simulink subsystem "ElectricMotorcycle"  (R2025b)
settings: Solver=VariableStepAuto  StartTime=0.0  StopTime=10.0  RelTol=1e-3
undefined symbols (not defined in the file): PlntDriveshftDamp, PlntDriveshftStiff, PlntEM1Damp, PlntEM1Inertia, PlntEM1Ratio
libraries: autolibsharedcoupling x2
settings Model: Creator=The MathWorks, Inc.  LastModifiedBy=The MathWorks, Inc.
settings RTWCC: GPUComputeCapability=3.5

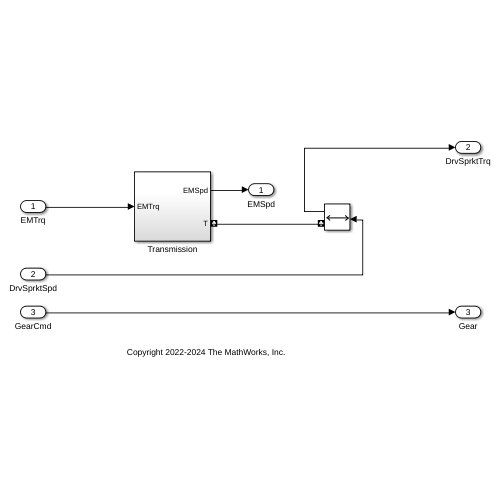
[thumbnail: Simulink's stored preview of the top-level diagram]
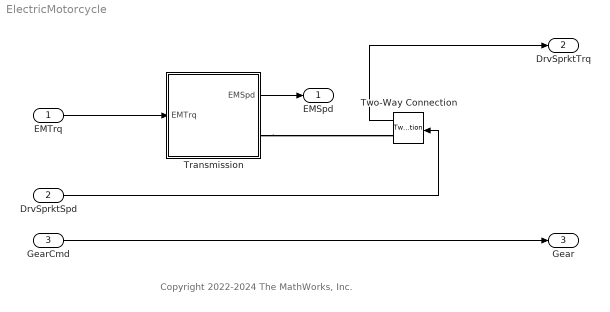
== system ElectricMotorcycle ==
  note: Copyright 2022-2024 The MathWorks, Inc.
  EMTrq : Inport
  DrvSprktSpd : Inport  Port=2
  GearCmd : Inport  Port=3
  Transmission : Subsystem
  Two-Way Connection : TwoWayConnection
  EMSpd : Outport  VectorParamsAs1DForOutWhenUnconnected=off  BusOutputAsStruct=on
  DrvSprktTrq : Outport  Port=2  VectorParamsAs1DForOutWhenUnconnected=off
  Gear : Outport  Port=3
  wires:
  Two-Way Connection/1 -> DrvSprktTrq/1
  Transmission/1(EMSpd) -> EMSpd/1
  EMTrq/1 -> Transmission/1(EMTrq)
  DrvSprktSpd/1 -> Two-Way Connection/1
  GearCmd/1 -> Gear/1
  connections:
  Transmission/RConn1 -- Two-Way Connection/RConn1

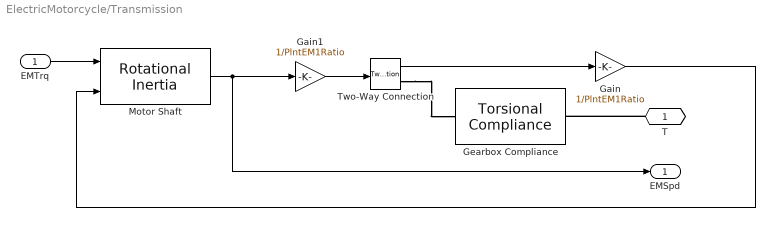
== system ElectricMotorcycle/Transmission ==
  EMTrq : Inport
  Gain : Gain  Gain=1/PlntEM1Ratio
  Gain1 : Gain  Gain=1/PlntEM1Ratio
  Gearbox Compliance : autolibsharedcoupling/Torsional Compliance  port_config=Two-way connection  extInfo=off  k=PlntDriveshftStiff  b=PlntDriveshftDamp  theta_o=PlntDriveshftInitDeflect  domega_o=PlntDriveshftInitVel  omega_c=PlntDriveshftDampCutoffFreq  blkID=0  aMode=6
  Motor Shaft : autolibsharedcoupling/Rotational Inertia  port_config=Simulink  extInfo=off  externJ=off  J=PlntEM1Inertia  b=PlntEM1Damp  omega_o=PlntEM1InitVel  blkID=0  aMode=6
      settings: LibrarySourceBlock=autolibcoupling/Rotational Inertia
  Two-Way Connection : TwoWayConnection
  T : PMIOPort  Side=Right
  EMSpd : Outport  VectorParamsAs1DForOutWhenUnconnected=off  BusOutputAsStruct=on
  wires:
  Gain1/1 -> Two-Way Connection/1
  Gain/1 -> Motor Shaft/2
  Two-Way Connection/1 -> Gain/1
  Motor Shaft/1 -> EMSpd/1, Gain1/1
  EMTrq/1 -> Motor Shaft/1
  connections:
  T/RConn1 -- Gearbox Compliance/RConn1
  Two-Way Connection/RConn1 -- Gearbox Compliance/LConn1
